simulink model "Calculator"  (R2018a)
settings: Solver=FixedStepDiscrete  StartTime=0.0  StopTime=10.0  RelTol=1e-3  EnableMultiTasking=on
settings Model: Creator=Fady  LastModifiedBy=Fady
settings OptimizationCC: DefaultParameterBehavior=Inlined  InlineInvariantSignals=on  EnableMemcpy=off  LifeSpan=1
settings DebuggingCC: UnderspecifiedInitializationDetection=Classic  MergeDetectMultiDrivingBlocksExec=none
settings ModelReferenceCC: PropagateSignalLabelsOutOfModel=off
settings SFSimCC: MATLABDynamicMemAlloc=off
settings RTWCC: SystemTargetFile=ert.tlc  GenCodeOnly=on  TemplateMakefile=ert_default_tmf  GenerateReport=on  IncludeHyperlinkInReport=on  LaunchReport=on  GenerateTraceInfo=on  GenerateTraceReport=on  GenerateTraceReportSl=on  GenerateTraceReportSf=on  GenerateTraceReportEml=on
settings CodeAppCC: ForceParamTrailComments=on  IgnoreCustomStorageClasses=off  OperatorAnnotations=on  SimulinkDataObjDesc=on  SFDataObjDesc=on  MATLABFcnDesc=on  InsertBlockDesc=on  StateflowObjectComments=on  MATLABSourceComments=on
settings ERTTargetCC: MultiwordLength=2048  GenerateSampleERTMain=on  InlinedParameterPlacement=NonHierarchical  ERTCustomFileTemplate=example_file_process.tlc

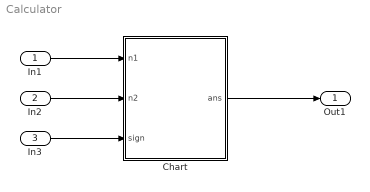
== system Calculator ==
  In1 : Inport  OutDataTypeStr=int8
  In2 : Inport  Port=2  OutDataTypeStr=int8
  In3 : Inport  Port=3  OutDataTypeStr=int8
  Chart : Stateflow chart  TreatAsAtomicUnit=on
  Out1 : Outport  OutDataTypeStr=int32
  wires:
  Chart/1(ans) -> Out1/1
  In1/1 -> Chart/1(n1)
  In2/1 -> Chart/2(n2)
  In3/1 -> Chart/3(sign)

== stateflow chart Calculator/Chart ==
  note: Do not put any code along
      | the transitions that run
      | down the right side!
  (default) -> (junction 25) : % calculator
  (junction 25) -> (junction 26) [order 1] : [sign == 0]
  (junction 25) -> (junction 29) [order 2]
  (junction 26) -> (junction 27) : {ans=n1+n2;}
  (junction 27) -> (junction 28)
  (junction 28) -> (junction 32)
  (junction 29) -> (junction 30) [order 1] : [sign == 1]
  (junction 29) -> (junction 33) [order 2]
  (junction 30) -> (junction 31) : {ans=n1-n2;}
  (junction 31) -> (junction 32)
  (junction 32) -> (junction 36)
  (junction 33) -> (junction 34) [order 1] : [sign == 2]
  (junction 33) -> (junction 37) [order 2]
  (junction 34) -> (junction 35) : {ans=n1*n2;}
  (junction 35) -> (junction 36)
  (junction 36) -> (junction 40)
  (junction 37) -> (junction 38) [order 1] : [sign == 3]
  (junction 37) -> (junction 43) [order 2]
  (junction 38) -> (junction 44) : [n2!=0]
  (junction 44) -> (junction 40) [order 1] : {ans=n1/n2}
  (junction 44) -> (junction 39) [order 2]
  (junction 39) -> (junction 40) : {ans=0;}
  (junction 40) -> (junction 42)
  (junction 42) -> ?
  data: ans output int32; n1 input int8; n2 input int8; sign input int8
